simulink model "calcula_trajetoria"  (R2017a)
settings: Solver=VariableStepAuto  StartTime=0.0  StopTime=15  RelTol=1e-3
libraries: simulink x6, UR3_Lib x1
settings Model: Creator=dscat  LastModifiedBy=dscat

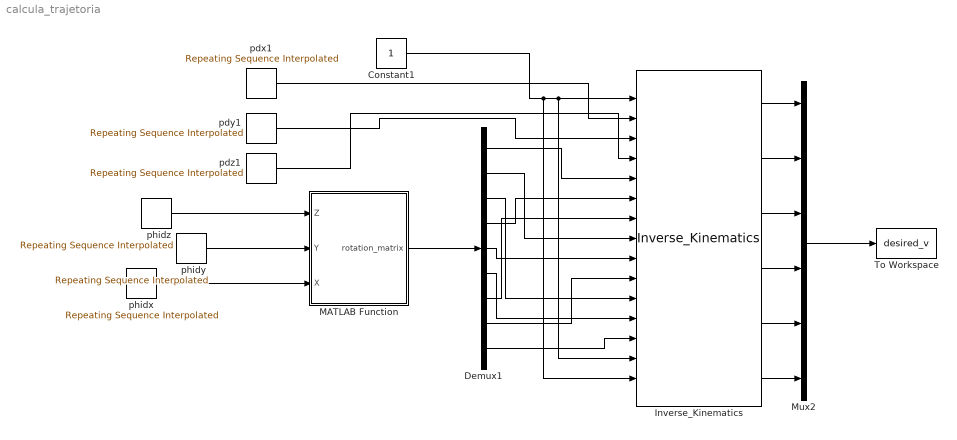
== system calcula_trajetoria ==
  Constant1 : Constant
  Demux1 : Demux  Outputs=9
  Inverse_Kinematics : UR3_Lib/Inverse_Kinematics
  MATLAB Function : MATLAB Function  TreatAsAtomicUnit=on
  Mux2 : Mux  Inputs=6
  To Workspace : ToWorkspace  VariableName=desired_v  SaveFormat=Timeseries  SampleTime=-1
  pdx1 : simulink/Sources/Repeating Sequence Interpolated  OutValues=pdx  TimeValues=t  LookUpMeth=Interpolation-Use End Values  tsamp=0.01  OutMin=[]  OutMax=[]  OutDataTypeStr=double  OutputDataTypeScalingMode=double  OutDataType=fixdt(0,8)  OutScaling=2^-10
  pdy1 : simulink/Sources/Repeating Sequence Interpolated  OutValues=pdy  TimeValues=t  LookUpMeth=Interpolation-Use End Values  tsamp=0.01  OutMin=[]  OutMax=[]  OutDataTypeStr=double  OutputDataTypeScalingMode=double  OutDataType=fixdt(0,8)  OutScaling=2^-10
  pdz1 : simulink/Sources/Repeating Sequence Interpolated  OutValues=pdz  TimeValues=t  LookUpMeth=Interpolation-Use End Values  tsamp=0.01  OutMin=[]  OutMax=[]  OutDataTypeStr=double  OutputDataTypeScalingMode=double  OutDataType=fixdt(0,8)  OutScaling=2^-10
  phidx : simulink/Sources/Repeating Sequence Interpolated  OutValues=phidx  TimeValues=t  LookUpMeth=Interpolation-Use End Values  tsamp=0.01  OutMin=[]  OutMax=[]  OutDataTypeStr=double  OutputDataTypeScalingMode=double  OutDataType=fixdt(0,8)  OutScaling=2^-10
  phidy : simulink/Sources/Repeating Sequence Interpolated  OutValues=phidy  TimeValues=t  LookUpMeth=Interpolation-Use End Values  tsamp=0.01  OutMin=[]  OutMax=[]  OutDataTypeStr=double  OutputDataTypeScalingMode=double  OutDataType=fixdt(0,8)  OutScaling=2^-10
  phidz : simulink/Sources/Repeating Sequence Interpolated  OutValues=phidz  TimeValues=t  LookUpMeth=Interpolation-Use End Values  tsamp=0.01  OutMin=[]  OutMax=[]  OutDataTypeStr=double  OutputDataTypeScalingMode=double  OutDataType=fixdt(0,8)  OutScaling=2^-10
  wires:
  phidz/1 -> MATLAB Function/1(Z)
  Inverse_Kinematics/2 -> Mux2/2
  Inverse_Kinematics/3 -> Mux2/3
  Inverse_Kinematics/1 -> Mux2/1
  Inverse_Kinematics/5 -> Mux2/5
  phidy/1 -> MATLAB Function/2(Y)
  Demux1/8 -> Inverse_Kinematics/10
  Inverse_Kinematics/6 -> Mux2/6
  Inverse_Kinematics/4 -> Mux2/4
  MATLAB Function/1(rotation_matrix) -> Demux1/1
  pdy1/1 -> Inverse_Kinematics/3
  Demux1/2 -> Inverse_Kinematics/8
  Constant1/1 -> Inverse_Kinematics/15, Inverse_Kinematics/14, Inverse_Kinematics/1
  phidx/1 -> MATLAB Function/3(X)
  Demux1/4 -> Inverse_Kinematics/6
  Demux1/5 -> Inverse_Kinematics/9
  Demux1/9 -> Inverse_Kinematics/13
  Demux1/6 -> Inverse_Kinematics/12
  Demux1/7 -> Inverse_Kinematics/7
  Demux1/1 -> Inverse_Kinematics/5
  pdz1/1 -> Inverse_Kinematics/4
  pdx1/1 -> Inverse_Kinematics/2
  Demux1/3 -> Inverse_Kinematics/11
  Mux2/1 -> To Workspace/1

== matlab function calcula_trajetoria/MATLAB Function ==
  data: Z input; rotation_matrix output; Y input; X input
function rotation_matrix = euler_rotationm(Z,Y,X)
eul = [Z X Y];
rotation_matrix = eul2rotm(eul);
